simulink model "excercise1_bd1"  (R2023b)
settings: Solver=VariableStepAuto  StartTime=0.0  StopTime=3  RelTol=1e-3
undefined symbols (not defined in the file): d, m
settings Model: Creator=elliot  LastModifiedBy=elliot

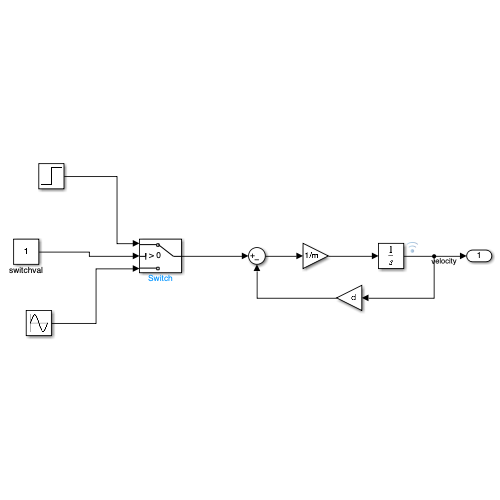
[thumbnail: Simulink's stored preview of the top-level diagram]
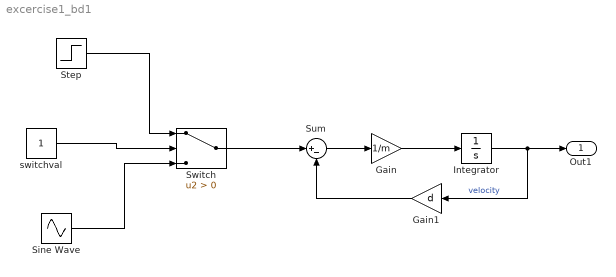
== system excercise1_bd1 ==
  Gain : Gain  Gain=1/m
  Gain1 : Gain  Gain=d
  Integrator : Integrator
  Sine Wave : Sin  SampleTime=0
  Step : Step  Time=0  SampleTime=0
  Sum : Sum  Inputs=|+-
  Switch : Switch  Criteria=u2 > Threshold  SaturateOnIntegerOverflow=off  InputSameDT=off
  switchval : Constant
  Out1 : Outport
  wires:
  Switch/1 -> Sum/1
  Step/1 -> Switch/1
  Sine Wave/1 -> Switch/3
  switchval/1 -> Switch/2
  Gain1/1 -> Sum/2
  Sum/1 -> Gain/1
  Gain/1 -> Integrator/1
  Integrator/1 -> Gain1/1, Out1/1  "velocity"
